simulink model "ur10_3DOF_regressor_control"  (Simulink 10.1)
settings: Solver=ode1  StartTime=0  StopTime=300  FixedStep=0.004  RelTol=1e-3  EnableMultiTasking=on
values from neighbouring files (symbols this model uses):
  anti_windup = ones(3, 1)    [TrajGen.m]    (also in anti_windup.m = abs(tau ./ joint_effort_limits) < 1)
undefined symbols (not defined in the file or in its folder): Dinamic_ur10_3DOF, ReferenceVelocity, SimpleRobotPlotROS, Tau, TrajGen
libraries: simulink x6
settings Model: Creator=E. Dean  LastModifiedBy=tard
settings Model: LogicAnalyzerGraphicalSettings=|
  | {
  |   "cursors" : {
  |     "activeCursor" : 0,
  |     "lockedCursors" : [
  | 
  |     ],
  |     "startingCursor" : 0,
  |     "times" : [
  |       0
  |     ]
  |   },
  |   "global" : {
  |   },
  |   "panels" : [
  |     {
  |       "height" : 100,
  |       "startingTrace" : 0,
  |       "traces" : [
  | 
  |       ],
  |       "yOffset" : 0
  |     }
  |   ],
  |   "timeAxis" : {
  |     "pixelsPerSecond" : 0.0000004930248214331365
  |   },
  |   "trigger" : {
  |     "enabled" : false,
  |     "mode" : "once",
  |     "samples" : 200,
  |     "signals" : {
  |     },
  |     "stages" : [
  |       {
  |         "conditions" : [
  | 
  |         ],
  |         "operator" : "AND"
  |       }
  |     ]
  |   }
  | }
settings DataIOCC: LimitDataPoints=on
settings OptimizationCC: ExpressionDepthLimit=2147483647
settings DebuggingCC: SolverPrmCheckMsg=warning  FcnCallInpInsideContextMsg=warning  AllowSymbolicDim=off  StateNameClashWarn=warning
settings ConfigComp: CovSFcnEnable=off

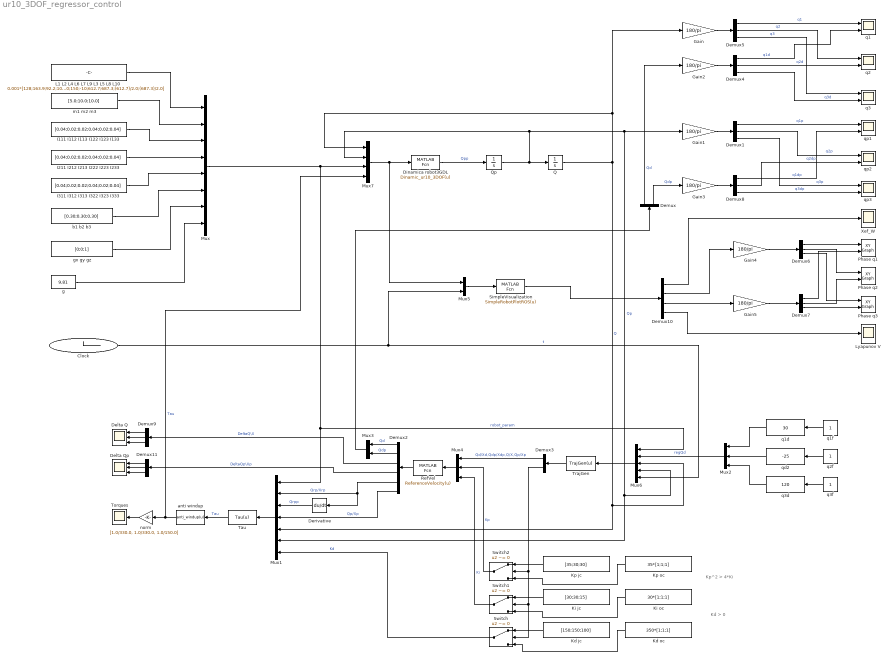
== system ur10_3DOF_regressor_control ==
  note: Kd > 0
  note: Kp^2 > 4*Ki
  Clock : Clock
  Delta Q : Scope  NumInputPorts=3
  Delta Qp : Scope  NumInputPorts=3
  Demux : Demux  Outputs=2
  Demux{1,4..9,11} (8 alike) : Demux  Outputs=3
  Demux10 : Demux  Outputs=[3 3 3 1]
  Demux2 : Demux  Outputs=6
  Demux3 : Demux  Outputs=[12 1]
  Derivative : Derivative
  Dinamica robot3GDL : MATLABFcn  MATLABFcn=Dinamic_ur10_3DOF(u)  OutputDimensions=3
  Gain{,1..5} (6 alike) : Gain  Gain=180/pi
  I111 I112 I113 I122 I123 I133 : Constant  Value=[0.04;0.02;0.02;0.04;0.02;0.04]
  I211 I212 I213 I222 I223 I233 : Constant  Value=[0.04;0.02;0.02;0.04;0.02;0.04]
  I311 I312 I313 I322 I323 I333 : Constant  Value=[0.04;0.02;0.02;0.04;0.02;0.04]
  "Kd jc " : Constant  Value=[150;150;100]
  Kd oc : Constant  Value=350*[1;1;1]
  Ki jc : Constant  Value=[30;30;15]
  Ki oc : Constant  Value=30*[1;1;1]
  Kp jc : Constant  Value=[35;30;30]
  Kp oc : Constant  Value=35*[1;1;1]
  "L1 L2 L4 L6 L7 L9 L3 L5 L8 L10 " : Constant  Value=0.001*[128;163.9;92.2;100;150;-10;612.7;687.3;(612.7)/2.0;(687.3)/2.0]  VectorParams1D=off
  Lyapunov V : Scope
  Mux : Mux  Inputs=8
  Mux1 : Mux  Inputs=7
  Mux2 : Mux  Inputs=3
  Mux3 : Mux  Inputs=2
  Mux4 : Mux  Inputs=3
  Mux5 : Mux  Inputs=2
  Mux6 : Mux  Inputs=5
  Mux7 : Mux
  Phase q1 : simulink/Sinks/XY Graph  xmin=-180  xmax=180  ymin=-3.5/pi*180  ymax=3.5/pi*180  st=-1
  Phase q2 : simulink/Sinks/XY Graph  xmin=-180  xmax=180  ymin=-3.5/pi*180  ymax=3.5/pi*180  st=-1
  Phase q3 : simulink/Sinks/XY Graph  xmin=-180  xmax=180  ymin=-3.5/pi*180  ymax=3.5/pi*180  st=-1
  Q : Integrator  InitialCondition=[0;0;0]
  Qp : Integrator  InitialCondition=[0;0;0]
  RefVel : MATLABFcn  MATLABFcn=ReferenceVelocity(u)  OutputDimensions=6*3
  SimpleVisualization : MATLABFcn  MATLABFcn=SimpleRobotPlotROS(u)  OutputDimensions=10
  Switch : Switch  Criteria=u2 ~= 0
  Switch1 : Switch  Criteria=u2 ~= 0
  Switch2 : Switch  Criteria=u2 ~= 0
  "Tau " : MATLABFcn  MATLABFcn=Tau(u)  OutputDimensions=3
  Torques : Scope
  TrajGen : MATLABFcn  MATLABFcn=TrajGen(u)  OutputDimensions=13
  Xef_W : Scope
  anti windup : MATLABFcn  MATLABFcn=anti_windup(u)  OutputDimensions=3
  "b1 b2 b3 " : Constant  Value=[0.30;0.30;0.30]
  g : Constant  Value=9.81
  gx gy gz : Constant  Value=[0;0;1]
  "m1 m2 m3 " : Constant  Value=[5.0;10.0;10.0]
  norm : Gain  Gain=[1.0/330.0, 1.0/330.0, 1.0/150.0]
  q1 : Scope  NumInputPorts=2
  q1d : simulink/Math Operations/Slider Gain  gain=30  low=-180  high=180
  q1f : Constant
  q2 : Scope  NumInputPorts=2
  q2f : Constant
  q3 : Scope  NumInputPorts=2
  q3d : simulink/Math Operations/Slider Gain  gain=120  low=-180  high=180
  q3f : Constant
  qd2 : simulink/Math Operations/Slider Gain  gain=-25  low=-180  high=180
  qp1 : Scope  NumInputPorts=2
  qp2 : Scope  NumInputPorts=2
  qp3 : Scope  NumInputPorts=2
  wires:
  Dinamica robot3GDL/1 -> Qp/1  "Qpp"
  Gain1/1 -> Demux1/1
  Demux1/1 -> qp1/1  "q1p"
  Demux1/2 -> qp2/1  "q2p"
  Demux1/3 -> qp3/1  "q3p"
  I111 I112 I113 I122 I123 I133/1 -> Mux/3
  I211 I212 I213 I222 I223 I233/1 -> Mux/4
  I311 I312 I313 I322 I323 I333/1 -> Mux/5
  Mux1/1 -> "Tau "/1
  q1f/1 -> q1d/1
  q2f/1 -> qd2/1
  q3f/1 -> q3d/1
  q1d/1 -> Mux2/1
  qd2/1 -> Mux2/2
  q3d/1 -> Mux2/3
  Q/1 -> Mux1/5, Mux6/3, Mux7/1, Gain/1  "Q"
  Qp/1 -> Gain1/1, Mux1/6, Mux6/4, Mux7/2, Q/1  "Qp"
  "m1 m2 m3 "/1 -> Mux/2
  "L1 L2 L4 L6 L7 L9 L3 L5 L8 L10 "/1 -> Mux/1
  Clock/1 -> Mux6/5, Mux5/2  "t"
  Demux4/1 -> q1/2  "q1d"
  Demux5/1 -> q1/1  "q1"
  Demux5/2 -> q2/1  "q2"
  Demux5/3 -> q3/1  "q3"
  Demux4/2 -> q2/2  "q2d"
  Demux4/3 -> q3/2  "q3d"
  Demux10/4 -> Lyapunov V/1
  Demux6/1 -> Phase q1/1
  Demux6/2 -> Phase q2/1
  Demux6/3 -> Phase q3/1
  Demux7/1 -> Phase q1/2
  Demux7/2 -> Phase q2/2
  Demux7/3 -> Phase q3/2
  Mux7/1 -> Mux5/1, Dinamica robot3GDL/1
  Mux/1 -> Mux1/1, Mux6/1, Mux7/3  "robot_param"
  Gain/1 -> Demux5/1
  Gain2/1 -> Demux4/1
  "b1 b2 b3 "/1 -> Mux/6
  gx gy gz/1 -> Mux/7
  g/1 -> Mux/8
  norm/1 -> Torques/1
  Derivative/1 -> Mux1/3  "Qrpp"
  RefVel/1 -> Demux2/1
  Demux2/5 -> Derivative/1, Mux1/2  "Qrp/Xrp"
  Gain3/1 -> Demux8/1
  Demux8/3 -> qp3/2  "q3dp"
  Demux8/2 -> qp2/2  "q2dp"
  Demux8/1 -> qp1/2  "q1dp"
  Demux2/1 -> Mux3/1  "Qd"
  Demux2/2 -> Mux3/2  "Qdp"
  Mux3/1 -> Demux/1
  Demux/1 -> Gain2/1  "Qd"
  Demux/2 -> Gain3/1  "Qdp"
  Mux4/1 -> RefVel/1
  Mux5/1 -> SimpleVisualization/1
  Mux6/1 -> TrajGen/1
  Mux2/1 -> Mux6/2  "regQd"
  anti windup/1 -> norm/1, Mux7/4  "Tau"
  "Tau "/1 -> anti windup/1  "Tau"
  Demux2/6 -> Mux1/4  "Qp/Xp"
  Demux10/2 -> Gain4/1
  Demux10/1 -> Xef_W/1
  SimpleVisualization/1 -> Demux10/1
  Gain4/1 -> Demux6/1
  Gain5/1 -> Demux7/1
  Demux10/3 -> Gain5/1
  Switch/1 -> Mux1/7  "Kd"
  "Kd jc "/1 -> Switch/1
  Kd oc/1 -> Switch/3
  Kp jc/1 -> Switch2/1
  Ki jc/1 -> Switch1/1
  Ki oc/1 -> Switch1/3
  Kp oc/1 -> Switch2/3
  Switch2/1 -> Mux4/2  "Kp"
  Switch1/1 -> Mux4/3  "Ki"
  TrajGen/1 -> Demux3/1
  Demux3/1 -> Mux4/1  "Qd/Xd,Qdp/Xdp,Q/X,Qp/Xp"
  Demux3/2 -> Switch1/2, Switch/2, Switch2/2
  Demux2/3 -> Demux9/1  "DeltaQ\\X"
  Demux9/1 -> Delta Q/1
  Demux9/2 -> Delta Q/2
  Demux9/3 -> Delta Q/3
  Demux11/2 -> Delta Qp/2
  Demux11/1 -> Delta Qp/1
  Demux11/3 -> Delta Qp/3
  Demux2/4 -> Demux11/1  "DeltaQp\\Xp"
